simulink model "SIMU_ROBOT"  (Simulink 8.1)
settings: Solver=ode45  StartTime=0.0  StopTime=inf  RelTol=1e-3
libraries: arduino_io_lib x11, simulink x5
settings Model: Creator=Usuario  LastModifiedBy=Usuario
settings DataIOCC: SignalLoggingSaveFormat=Dataset
settings OptimizationCC: ExpressionDepthLimit=128
settings DebuggingCC: FcnCallInpInsideContextMsg=EnableAllAsError
settings GRTTargetCC: CombineOutputUpdateFcns=on  GRTInterface=off
settings ConfigurationSet: Description=SimMechanics 2G

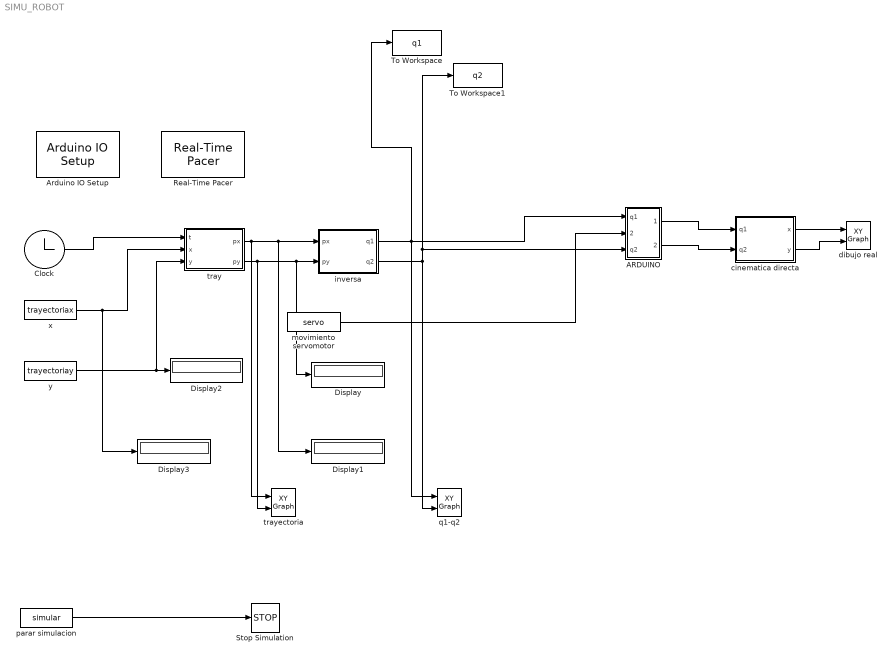
== system SIMU_ROBOT ==
  "ARDUINO " : Subsystem
  Arduino IO Setup : arduino_io_lib/Arduino IO Setup  Priority=3  arduinoVar=Temporary arduino variable: Arduino1  workspaceVarName=a  comPort=COM4
  Clock : Clock
  Display{,1..3} (4 alike) : Display
  Real-Time Pacer : arduino_io_lib/Real-Time Pacer  simTimePerRealTime=1
  Stop Simulation : Stop
  To Workspace : ToWorkspace  VariableName=q1  SampleTime=-1  SaveFormat=Timeseries
  To Workspace1 : ToWorkspace  VariableName=q2  SampleTime=-1  SaveFormat=Timeseries
  cinematica directa : MATLAB Function  TreatAsAtomicUnit=on
  dibujo real : simulink/Sinks/XY Graph  xmin=-20  xmax=40  ymin=-30  ymax=30  st=-1
  inversa : MATLAB Function  TreatAsAtomicUnit=on
  movimiento servomotor : FromWorkspace  VariableName=servo  SampleTime=1  Interpolate=off  OutputAfterFinalValue=Holding final value
  "parar simulacion " : FromWorkspace  VariableName=simular  SampleTime=0  OutputAfterFinalValue=Holding final value
  "q1-q2 " : simulink/Sinks/XY Graph  xmin=-20  xmax=20  ymin=-20  ymax=20  st=-1
  tray : MATLAB Function  TreatAsAtomicUnit=on
  trayectoria : simulink/Sinks/XY Graph  xmin=0  xmax=40  ymin=-20  ymax=20  st=-1
  x : FromWorkspace  VariableName=trayectoriax  SampleTime=1  Interpolate=off  OutputAfterFinalValue=Holding final value
  y : FromWorkspace  VariableName=trayectoriay  SampleTime=0  OutputAfterFinalValue=Holding final value
  wires:
  x/1 -> Display3/1, tray/2(x)
  y/1 -> Display2/1, tray/3(y)
  Clock/1 -> tray/1(t)
  tray/1(px) -> Display1/1, inversa/1(px), trayectoria/1
  tray/2(py) -> Display/1, inversa/2(py), trayectoria/2
  inversa/2(q2) -> "ARDUINO "/3(q2), To Workspace1/1, "q1-q2 "/2
  inversa/1(q1) -> To Workspace/1, "ARDUINO "/1(q1), "q1-q2 "/1
  "parar simulacion "/1 -> Stop Simulation/1
  movimiento servomotor/1 -> "ARDUINO "/2(servo)
  "ARDUINO "/1(Out1) -> cinematica directa/1(q1)
  "ARDUINO "/2(Out2) -> cinematica directa/2(q2)
  cinematica directa/1(x) -> dibujo real/1
  cinematica directa/2(y) -> dibujo real/2

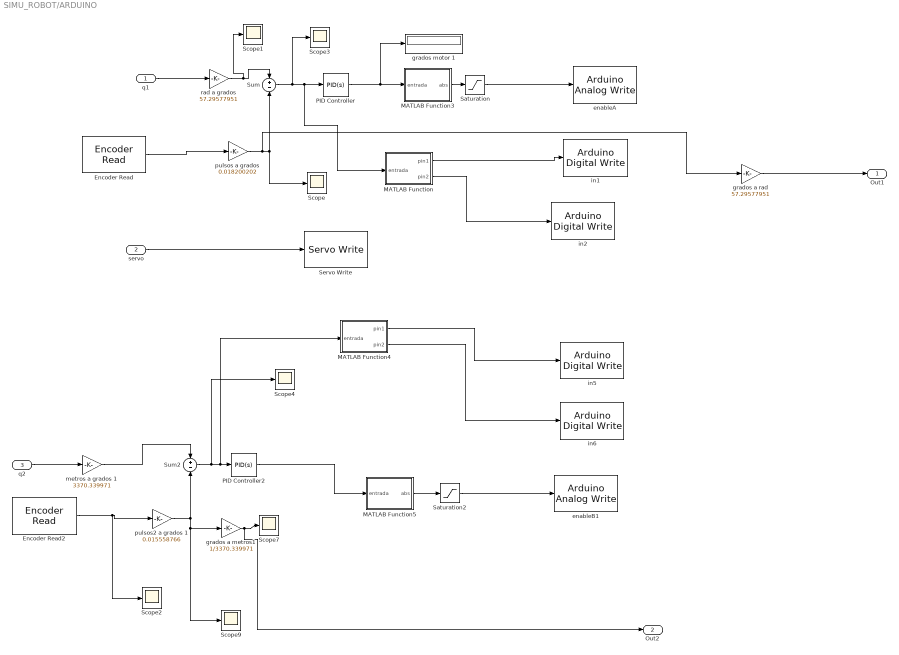
== system SIMU_ROBOT/ARDUINO  ==
  q1 : Inport
  servo : Inport  Port=2
  q2 : Inport  Port=3
  Encoder Read : arduino_io_lib/Encoder Read  arduinoVar=Temporary arduino variable: Arduino1  encNum=1  pinA=19  pinB=18  DbDl=0  T=0.2
  Encoder Read2 : arduino_io_lib/Encoder Read  arduinoVar=Temporary arduino variable: Arduino1  encNum=2  pinA=21  pinB=20  DbDl=0  T=0.2
  MATLAB Function : MATLAB Function  TreatAsAtomicUnit=on
  MATLAB Function3 : MATLAB Function  TreatAsAtomicUnit=on
  MATLAB Function4 : MATLAB Function  TreatAsAtomicUnit=on
  MATLAB Function5 : MATLAB Function  TreatAsAtomicUnit=on
  PID Controller : simulink/Continuous/PID Controller  Controller=PID  TimeDomain=Continuous-time  SampleTime=1  IntegratorMethod=Forward Euler  FilterMethod=Forward Euler  Form=Parallel  P=300  I=3000  D=75  N=100  InitialConditionSource=internal  InitialConditionForIntegrator=0  InitialConditionForFilter=0  ExternalReset=none  LimitOutput=off  UpperSaturationLimit=inf  LowerSaturationLimit=-inf  LinearizeAsGain=on  AntiWindupMode=none  Kb=1  TrackingMode=off  Kt=1  PParamMin=[]  PParamMax=[]  IParamMin=[]  IParamMax=[]  DParamMin=[]  DParamMax=[]  NParamMin=[]  NParamMax=[]  KbParamMin=[]  KbParamMax=[]  KtParamMin=[]  KtParamMax=[]  POutMin=[]  POutMax=[]  IOutMin=[]  IOutMax=[]  DOutMin=[]  DOutMax=[]  NOutMin=[]  NOutMax=[]  KbOutMin=[]  KbOutMax=[]  KtOutMin=[]  KtOutMax=[]  IntegratorOutMin=[]  IntegratorOutMax=[]  FilterOutMin=[]  FilterOutMax=[]  SumOutMin=[]  SumOutMax=[]  SumI1OutMin=[]  SumI1OutMax=[]  SumI2OutMin=[]  SumI2OutMax=[]  SumI3OutMin=[]  SumI3OutMax=[]  SumDOutMin=[]  SumDOutMax=[]  SaturationOutMin=[]  SaturationOutMax=[]  IntegratorContinuousStateAttributes=''  IntegratorStateMustResolveToSignalObject=off  IntegratorRTWStateStorageClass=Auto  FilterContinuousStateAttributes=''  FilterStateMustResolveToSignalObject=off  FilterRTWStateStorageClass=Auto
  PID Controller2 : simulink/Continuous/PID Controller  Controller=PID  TimeDomain=Continuous-time  SampleTime=1  IntegratorMethod=Forward Euler  FilterMethod=Forward Euler  Form=Parallel  P=42  I=53  D=9  N=100  InitialConditionSource=internal  InitialConditionForIntegrator=0  InitialConditionForFilter=0  ExternalReset=none  LimitOutput=off  UpperSaturationLimit=inf  LowerSaturationLimit=-inf  LinearizeAsGain=on  AntiWindupMode=none  Kb=1  TrackingMode=off  Kt=1  PParamMin=[]  PParamMax=[]  IParamMin=[]  IParamMax=[]  DParamMin=[]  DParamMax=[]  NParamMin=[]  NParamMax=[]  KbParamMin=[]  KbParamMax=[]  KtParamMin=[]  KtParamMax=[]  POutMin=[]  POutMax=[]  IOutMin=[]  IOutMax=[]  DOutMin=[]  DOutMax=[]  NOutMin=[]  NOutMax=[]  KbOutMin=[]  KbOutMax=[]  KtOutMin=[]  KtOutMax=[]  IntegratorOutMin=[]  IntegratorOutMax=[]  FilterOutMin=[]  FilterOutMax=[]  SumOutMin=[]  SumOutMax=[]  SumI1OutMin=[]  SumI1OutMax=[]  SumI2OutMin=[]  SumI2OutMax=[]  SumI3OutMin=[]  SumI3OutMax=[]  SumDOutMin=[]  SumDOutMax=[]  SaturationOutMin=[]  SaturationOutMax=[]  IntegratorContinuousStateAttributes=''  IntegratorStateMustResolveToSignalObject=off  IntegratorRTWStateStorageClass=Auto  FilterContinuousStateAttributes=''  FilterStateMustResolveToSignalObject=off  FilterRTWStateStorageClass=Auto
  Saturation : Saturate  UpperLimit=255  LowerLimit=0
  Saturation2 : Saturate  UpperLimit=255  LowerLimit=0
  Scope{,1..4,7,9} (7 alike) : Scope
      Scope2 settings: SaveName=ScopeData4
      Scope3 settings: SaveName=ScopeData3
      Scope4 settings: SaveName=ScopeData5
      Scope7 settings: SaveName=ScopeData6
      Scope9 settings: SaveName=ScopeData7
  Servo Write : arduino_io_lib/Servo Write  arduinoVar=Temporary arduino variable: Arduino1  pinNum=8  T=0.2
  Sum : Sum  Inputs=+-
  Sum2 : Sum  Inputs=+-
  enableA : arduino_io_lib/Arduino Analog Write  arduinoVar=Temporary arduino variable: Arduino1  arduinoPin=6  T=0.2
  enableB1 : arduino_io_lib/Arduino Analog Write  arduinoVar=Temporary arduino variable: Arduino1  arduinoPin=5  T=0.2
  grados a metros1 : Gain  Gain=1/3370.339971
  grados a rad : Gain  Gain=57.29577951
  "grados motor 1 " : Display
  in1 : arduino_io_lib/Arduino Digital Write  arduinoVar=Temporary arduino variable: Arduino1  arduinoPin=7  T=0.2
  in2 : arduino_io_lib/Arduino Digital Write  arduinoVar=Temporary arduino variable: Arduino1  arduinoPin=4  T=0.2
  in5 : arduino_io_lib/Arduino Digital Write  arduinoVar=Temporary arduino variable: Arduino1  arduinoPin=3  T=0.2
  in6 : arduino_io_lib/Arduino Digital Write  arduinoVar=Temporary arduino variable: Arduino1  arduinoPin=2  T=0.2
  metros a grados 1 : Gain  Gain=3370.339971
  pulsos a grados : Gain  Gain=0.018200202
  pulsos2 a grados 1 : Gain  Gain=0.015558766
  "rad a grados " : Gain  Gain=57.29577951
  Out1 : Outport
  Out2 : Outport  Port=2
  wires:
  q1/1 -> "rad a grados "/1
  pulsos a grados/1 -> grados a rad/1, Sum/2, Scope/1
  Encoder Read/1 -> pulsos a grados/1
  "rad a grados "/1 -> Scope1/1, Sum/1
  Sum/1 -> Scope3/1, MATLAB Function/1(entrada), PID Controller/1
  PID Controller/1 -> MATLAB Function3/1(entrada), "grados motor 1 "/1
  MATLAB Function/1(pin1) -> in1/1
  MATLAB Function/2(pin2) -> in2/1
  Saturation/1 -> enableA/1
  servo/1 -> Servo Write/1
  MATLAB Function3/1(abs) -> Saturation/1
  Encoder Read2/1 -> Scope2/1, pulsos2 a grados 1/1
  pulsos2 a grados 1/1 -> Sum2/2, Scope9/1, grados a metros1/1
  metros a grados 1/1 -> Sum2/1
  Sum2/1 -> Scope4/1, MATLAB Function4/1(entrada), PID Controller2/1
  PID Controller2/1 -> MATLAB Function5/1(entrada)
  MATLAB Function4/1(pin1) -> in5/1
  MATLAB Function4/2(pin2) -> in6/1
  Saturation2/1 -> enableB1/1
  MATLAB Function5/1(abs) -> Saturation2/1
  q2/1 -> metros a grados 1/1
  grados a rad/1 -> Out1/1
  grados a metros1/1 -> Out2/1, Scope7/1

== matlab function inversa ==
  data: px input double; py input double; q1 output double; q2 output double
function [q1,q2]= fcn(px,py)
%#codegen

q1=atan2(py,px);
q2=(cos(q1)*px+sin(q1)*py-9.7)/100;

== matlab function tray ==
  data: t input double; x input double; y input double; px output double; py output double
function [px,py]= fcn(t,x,y)
%#codegen

px=x;
py=y;

== matlab function ARDUINO /MATLAB Function ==
  data: entrada input double; pin1 output double; pin2 output double
function [pin1,pin2] = fcn(entrada)

if(entrada>0)
    pin1=1;
    pin2=0;
else
    pin1=0;
    pin2=1;
end

== matlab function cinematica directa ==
  data: q1 input double; q2 input double; x output double; y output double
function [x,y]= fcn(q1,q2)
%#codegen

x=(cos(q1)*(0.097+q2))*100;
y=(sin(q1)*(0.097+q2))*100;

== matlab function ARDUINO /MATLAB Function3 ==
  data: entrada input double; abs output double
function abs  = fcn(entrada)

if(entrada<0)
    abs=entrada*(-1);
else
    abs=entrada;
end

== matlab function ARDUINO /MATLAB Function4 ==
  data: entrada input double; pin1 output double; pin2 output double
function [pin1,pin2] = fcn(entrada)

if(entrada>0)
    pin1=1;
    pin2=0;
else
    pin1=0;
    pin2=1;
end

== matlab function ARDUINO /MATLAB Function5 ==
  data: entrada input double; abs output double
function abs  = fcn(entrada)

if(entrada<0)
    abs=entrada*(-1);
else
    abs=entrada;
end
